simulink library "IPT_lib"  (Simulink 7.4)
settings: Solver=ode45  StartTime=0.0  StopTime=10.0  RelTol=1e-3
values from neighbouring files (symbols this model uses):
  IPTa_i_ShuntCur = mpt.Parameter    [IPT_ANALOG_CAL.m]
  IPTc_Gain_KL30 = mpt.Parameter    [IPT_ANALOG_CAL.m]
  IPTc_Gain_MSDVolt = mpt.Parameter    [IPT_ANALOG_CAL.m]
  IPTc_Gain_PCBTemp = mpt.Parameter    [IPT_ANALOG_CAL.m]
  IPTc_Gain_PosCtrVoltRef1_back = mpt.Parameter    [IPT_ANALOG_CAL.m]
  IPTc_Gain_PosCtrVoltRef1_front = mpt.Parameter    [IPT_ANALOG_CAL.m]
  IPTc_Gain_PosCtrVoltRef2_back = mpt.Parameter    [IPT_ANALOG_CAL.m]
  IPTc_Gain_PosCtrVoltRef2_front = mpt.Parameter    [IPT_ANALOG_CAL.m]
  IPTc_pct_CellInitSoc = mpt.Parameter    [IPT_INTERNAL_CAL.m]
  IPTc_t_BMUInitTemp = mpt.Parameter    [IPT_CAN_CAL.m]
  IPTc_t_MdlInitTemp = mpt.Parameter    [IPT_CAN_CAL.m]
  IPTc_t_PCBTemp_max = mpt.Parameter    [IPT_ANALOG_CAL.m]
  IPTc_t_PCBTemp_min = mpt.Parameter    [IPT_ANALOG_CAL.m]
  IPTc_v_KL30_max = mpt.Parameter    [IPT_ANALOG_CAL.m]
  IPTc_v_KL30_min = mpt.Parameter    [IPT_ANALOG_CAL.m]
  IPTc_v_MSDVolt_max = mpt.Parameter    [IPT_ANALOG_CAL.m]
  IPTc_v_MSDVolt_min = mpt.Parameter    [IPT_ANALOG_CAL.m]
  IPTc_v_PosCtrVoltRef1_back_max = mpt.Parameter    [IPT_ANALOG_CAL.m]
  IPTc_v_PosCtrVoltRef1_back_min = mpt.Parameter    [IPT_ANALOG_CAL.m]
  IPTc_v_PosCtrVoltRef1_front_max = mpt.Parameter    [IPT_ANALOG_CAL.m]
  IPTc_v_PosCtrVoltRef1_front_min = mpt.Parameter    [IPT_ANALOG_CAL.m]
  IPTc_v_PosCtrVoltRef2_back_max = mpt.Parameter    [IPT_ANALOG_CAL.m]
  IPTc_v_PosCtrVoltRef2_back_min = mpt.Parameter    [IPT_ANALOG_CAL.m]
  IPTc_v_PosCtrVoltRef2_front_max = mpt.Parameter    [IPT_ANALOG_CAL.m]
  IPTc_v_PosCtrVoltRef2_front_min = mpt.Parameter    [IPT_ANALOG_CAL.m]
  IPTf_fac_ShuntCurCorrect = mpt.Parameter    [IPT_ANALOG_CAL.m]
undefined symbols (not defined in the file or in its folder): CTC_DriveOnline_St, CTC_FastChaOnline_St, CTC_SlowChaOnline_St, IPTa_v_PCBTemp, IPTc_Gain_BMUPowSplyCur, IPTc_Gain_ShuntCur, IPTc_Gain_USample, IPTc_i_BMUPowSplyCur_max, IPTc_i_BMUPowSplyCur_min, IPTc_i_ShuntCur_max, IPTc_i_ShuntCur_min, IPTc_v_CC2_OffDnLimit, IPTc_v_CC2_OffUpLimit, IPTc_v_CC2_OnDnLimit, IPTc_v_CC2_OnUpLimit, IPTc_v_CellInitVolt, IPTc_v_SlowChalineCnctStLowLimFir, IPTc_v_SlowChalineCnctStLowLimSec, IPTc_v_SlowChalineCnctStUppLimFir, IPTc_v_SlowChalineCnctStUppLimSec, IPTc_v_SlowChalineOpenLowLim, IPTc_v_SlowChalineOpenUppLim, IPTc_v_USample_max, IPTc_v_USample_min, IPTf_t_PCBTemp, PACK_Const_BMUNumOfPack
libraries: Defined_Functionality x129
(part 1 of 3)
settings Model: Creator=zhangyanqiao  LastModifiedBy=zhouping

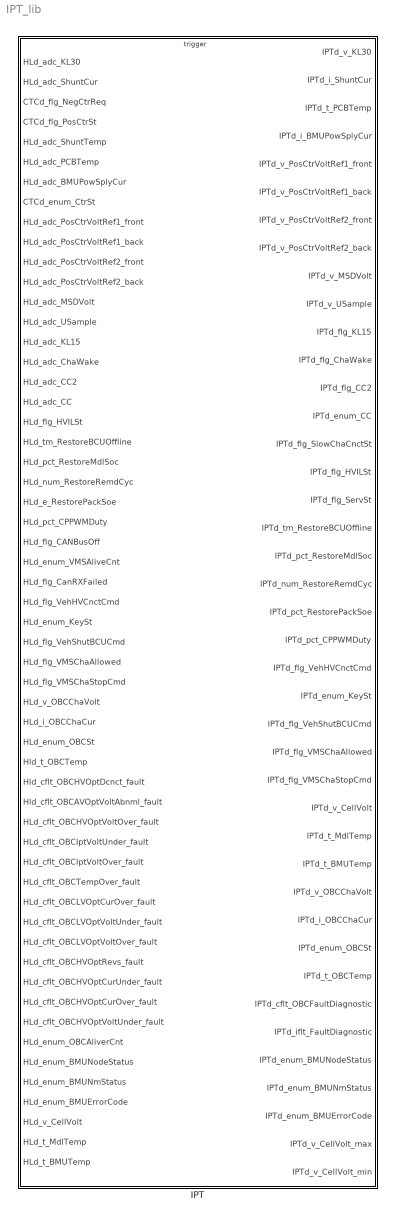
== system IPT_lib ==
  IPT : Subsystem  TreatAsAtomicUnit=on  RTWFcnName=IPT
      settings: RTWFileNameOpts=Use function name

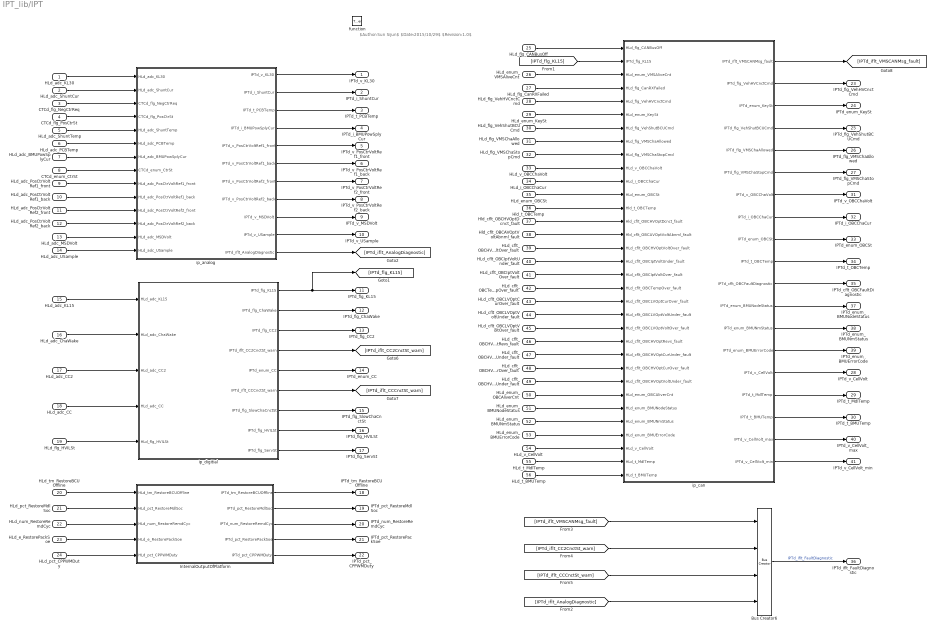
== system IPT_lib/IPT ==
  note: $Author:Sun Sijun$
      | $Date:2015/10/29$
      | $Revision:1.0$
  HLd_adc_KL30 : Inport
  HLd_adc_ShuntCur : Inport  Port=2
  CTCd_flg_NegCtrReq : Inport  Port=3
  CTCd_flg_PosCtrSt : Inport  Port=4
  HLd_adc_ShuntTemp : Inport  Port=5
  HLd_adc_PCBTemp : Inport  Port=6
  HLd_adc_BMUPowSplyCur : Inport  Port=7
  CTCd_enum_CtrSt : Inport  Port=8
  HLd_adc_PosCtrVoltRef1_front : Inport  Port=9
  HLd_adc_PosCtrVoltRef1_back : Inport  Port=10
  HLd_adc_PosCtrVoltRef2_front : Inport  Port=11
  HLd_adc_PosCtrVoltRef2_back : Inport  Port=12
  HLd_adc_MSDVolt : Inport  Port=13
  HLd_adc_USample : Inport  Port=14  OutDataType=fixdt(1, 16)  OutScaling=2^0
  HLd_adc_KL15 : Inport  Port=15
  HLd_adc_ChaWake : Inport  Port=16  OutDataType=fixdt(1, 16)  OutScaling=2^0
  HLd_adc_CC2 : Inport  Port=17  OutDataType=fixdt(1, 16)  OutScaling=2^0
  HLd_adc_CC : Inport  Port=18  OutDataType=fixdt(1, 16)  OutScaling=2^0
  HLd_flg_HVILSt : Inport  Port=19  OutDataType=fixdt(1, 16)  OutScaling=2^0
  HLd_tm_RestoreBCUOffline : Inport  Port=20  OutDataType=fixdt(1, 16)  OutScaling=2^0
  HLd_pct_RestoreMdlSoc : Inport  Port=21  OutDataType=fixdt(1, 16)  OutScaling=2^0
  HLd_num_RestoreRemdCyc : Inport  Port=22  OutDataType=fixdt(1, 16)  OutScaling=2^0
  HLd_e_RestorePackSoe : Inport  Port=23  OutDataType=fixdt(1, 16)  OutScaling=2^0
  HLd_pct_CPPWMDuty : Inport  Port=24  OutDataType=fixdt(1, 16)  OutScaling=2^0
  HLd_flg_CANBusOff : Inport  Port=25
  HLd_enum_VMSAliveCnt : Inport  Port=26  OutDataType=fixdt(1, 16)  OutScaling=2^0
  HLd_flg_CanRXFailed : Inport  Port=27  OutDataType=fixdt(1, 16)  OutScaling=2^0
  HLd_flg_VehHVCnctCmd : Inport  Port=28  OutDataType=fixdt(1, 16)  OutScaling=2^0
  HLd_enum_KeySt : Inport  Port=29  OutDataType=fixdt(1, 16)  OutScaling=2^0
  HLd_flg_VehShutBCUCmd : Inport  Port=30  OutDataType=fixdt(1, 16)  OutScaling=2^0
  HLd_flg_VMSChaAllowed : Inport  Port=31  OutDataType=fixdt(1, 16)  OutScaling=2^0
  HLd_flg_VMSChaStopCmd : Inport  Port=32  OutDataType=fixdt(1, 16)  OutScaling=2^0
  HLd_v_OBCChaVolt : Inport  Port=33
  HLd_i_OBCChaCur : Inport  Port=34
  HLd_enum_OBCSt : Inport  Port=35
  Hld_t_OBCTemp : Inport  Port=36
  Hld_cflt_OBCHVOptDcnct_fault : Inport  Port=37
  Hld_cflt_OBCAVOptVoltAbnml_fault : Inport  Port=38
  HLd_cflt_OBCHVOptVoltOver_fault : Inport  Port=39
  HLd_cflt_OBCIptVoltUnder_fault : Inport  Port=40
  HLd_cflt_OBCIptVoltOver_fault : Inport  Port=41
  HLd_cflt_OBCTempOver_fault : Inport  Port=42
  HLd_cflt_OBCLVOptCurOver_fault : Inport  Port=43
  HLd_cflt_OBCLVOptVoltUnder_fault : Inport  Port=44
  HLd_cflt_OBCLVOptVoltOver_fault : Inport  Port=45
  HLd_cflt_OBCHVOptRevs_fault : Inport  Port=46
  HLd_cflt_OBCHVOptCurUnder_fault : Inport  Port=47
  HLd_cflt_OBCHVOptCurOver_fault : Inport  Port=48
  HLd_cflt_OBCHVOptVoltUnder_fault : Inport  Port=49
  HLd_enum_OBCAliverCnt : Inport  Port=50
  HLd_enum_BMUNodeStatus : Inport  Port=51
  HLd_enum_BMUNmStatus : Inport  Port=52
  HLd_enum_BMUErrorCode : Inport  Port=53
  HLd_v_CellVolt : Inport  Port=54
  HLd_t_MdlTemp : Inport  Port=55
  HLd_t_BMUTemp : Inport  Port=56
  function : TriggerPort  TriggerType=function-call
  Bus Creator6 : BusCreator
  InternalOutputOfPlatform : Subsystem
  ip_analog : Subsystem  Description=$Author:Zhao XiangRi$
  ip_can : Subsystem
  ip_digitial : Subsystem
  IPTd_v_KL30 : Outport
  IPTd_i_ShuntCur : Outport  Port=2
  IPTd_t_PCBTemp : Outport  Port=3
  IPTd_i_BMUPowSplyCur : Outport  Port=4
  IPTd_v_PosCtrVoltRef1_front : Outport  Port=5
  IPTd_v_PosCtrVoltRef1_back : Outport  Port=6
  IPTd_v_PosCtrVoltRef2_front : Outport  Port=7
  IPTd_v_PosCtrVoltRef2_back : Outport  Port=8
  IPTd_v_MSDVolt : Outport  Port=9
  IPTd_v_USample : Outport  Port=10
  IPTd_flg_KL15 : Outport  Port=11  OutDataType=fixdt(1, 16)  OutScaling=2^0
  IPTd_flg_ChaWake : Outport  Port=12  OutDataType=fixdt(1, 16)  OutScaling=2^0
  IPTd_flg_CC2 : Outport  Port=13  OutDataType=fixdt(1, 16)  OutScaling=2^0
  IPTd_enum_CC : Outport  Port=14  OutDataType=fixdt(1, 16)  OutScaling=2^0
  IPTd_flg_SlowChaCnctSt : Outport  Port=15  OutDataType=fixdt(1, 16)  OutScaling=2^0
  IPTd_flg_HVILSt : Outport  Port=16  OutDataType=fixdt(1, 16)  OutScaling=2^0
  IPTd_flg_ServSt : Outport  Port=17  OutDataType=fixdt(1, 16)  OutScaling=2^0
  IPTd_tm_RestoreBCUOffline : Outport  Port=18  OutDataType=fixdt(1, 16)  OutScaling=2^0
  IPTd_pct_RestoreMdlSoc : Outport  Port=19  OutDataType=fixdt(1, 16)  OutScaling=2^0
  IPTd_num_RestoreRemdCyc : Outport  Port=20  OutDataType=fixdt(1, 16)  OutScaling=2^0
  IPTd_pct_RestorePackSoe : Outport  Port=21  OutDataType=fixdt(1, 16)  OutScaling=2^0
  IPTd_pct_CPPWMDuty : Outport  Port=22  OutDataType=fixdt(1, 16)  OutScaling=2^0
  IPTd_flg_VehHVCnctCmd : Outport  Port=23  OutDataType=fixdt(1, 16)  OutScaling=2^0
  IPTd_enum_KeySt : Outport  Port=24  OutDataType=fixdt(1, 16)  OutScaling=2^0
  IPTd_flg_VehShutBCUCmd : Outport  Port=25  OutDataType=fixdt(1, 16)  OutScaling=2^0
  IPTd_flg_VMSChaAllowed : Outport  Port=26  OutDataType=fixdt(1, 16)  OutScaling=2^0
  IPTd_flg_VMSChaStopCmd : Outport  Port=27  OutDataType=fixdt(1, 16)  OutScaling=2^0
  IPTd_v_CellVolt : Outport  Port=28
  IPTd_t_MdlTemp : Outport  Port=29
  IPTd_t_BMUTemp : Outport  Port=30
  IPTd_v_OBCChaVolt : Outport  Port=31
  IPTd_i_OBCChaCur : Outport  Port=32
  IPTd_enum_OBCSt : Outport  Port=33
  IPTd_t_OBCTemp : Outport  Port=34
  IPTd_cflt_OBCFaultDiagnostic : Outport  Port=35
  IPTd_iflt_FaultDiagnostic : Outport  Port=36
  "IPTd_enum_BMUNodeStatus " : Outport  Port=37
  IPTd_enum_BMUNmStatus : Outport  Port=38
  IPTd_enum_BMUErrorCode : Outport  Port=39
  IPTd_v_CellVolt_max : Outport  Port=40
  IPTd_v_CellVolt_min : Outport  Port=41
  wires:
  ip_can/19(IPTd_v_CellVolt_min) -> IPTd_v_CellVolt_min/1
  ip_can/18(IPTd_v_CellVolt_max) -> IPTd_v_CellVolt_max/1
  [IPTd_iflt_CCCnctSt_warn] -> Bus Creator6/3
  [IPTd_iflt_CC2CnctSt_warn] -> Bus Creator6/2
  ip_can/10(IPTd_t_OBCTemp) -> IPTd_t_OBCTemp/1
  Hld_cflt_OBCAVOptVoltAbnml_fault/1 -> ip_can/15(Hld_cflt_OBCAVOptVoltAbnml_fault)
  Hld_cflt_OBCHVOptDcnct_fault/1 -> ip_can/14(Hld_cflt_OBCHVOptDcnct_fault)
  Hld_t_OBCTemp/1 -> ip_can/13(Hld_t_OBCTemp)
  CTCd_flg_PosCtrSt/1 -> ip_analog/4(CTCd_flg_PosCtrSt)
  CTCd_flg_NegCtrReq/1 -> ip_analog/3(CTCd_flg_NegCtrReq)
  CTCd_enum_CtrSt/1 -> ip_analog/8(CTCd_enum_CtrSt)
  ip_digitial/9(IPTd_flg_ServSt) -> IPTd_flg_ServSt/1
  HLd_enum_BMUErrorCode/1 -> ip_can/30(HLd_enum_BMUErrorCode)
  HLd_enum_BMUNmStatus/1 -> ip_can/29(HLd_enum_BMUNmStatus)
  HLd_enum_BMUNodeStatus/1 -> ip_can/28(HLd_enum_BMUNodeStatus)
  ip_can/14(IPTd_enum_BMUErrorCode) -> IPTd_enum_BMUErrorCode/1
  ip_can/13(IPTd_enum_BMUNmStatus) -> IPTd_enum_BMUNmStatus/1
  ip_can/12("IPTd_enum_BMUNodeStatus ") -> "IPTd_enum_BMUNodeStatus "/1
  [IPTd_iflt_AnalogDiagnostic] -> Bus Creator6/4
  ip_analog/11(IPTd_iflt_AnalogDiagnostic) -> [IPTd_iflt_AnalogDiagnostic]
  ip_analog/8(IPTd_v_PosCtrVoltRef2_back) -> IPTd_v_PosCtrVoltRef2_back/1
  ip_analog/7(IPTd_v_PosCtrVoltRef2_front) -> IPTd_v_PosCtrVoltRef2_front/1
  ip_analog/6(IPTd_v_PosCtrVoltRef1_back) -> IPTd_v_PosCtrVoltRef1_back/1
  ip_analog/5(IPTd_v_PosCtrVoltRef1_front) -> IPTd_v_PosCtrVoltRef1_front/1
  ip_digitial/7(IPTd_flg_SlowChaCnctSt) -> IPTd_flg_SlowChaCnctSt/1
  ip_can/17(IPTd_t_BMUTemp) -> IPTd_t_BMUTemp/1
  HLd_t_BMUTemp/1 -> ip_can/33(HLd_t_BMUTemp)
  ip_can/11(IPTd_cflt_OBCFaultDiagnostic) -> IPTd_cflt_OBCFaultDiagnostic/1
  ip_can/9(IPTd_enum_OBCSt) -> IPTd_enum_OBCSt/1
  ip_can/8(IPTd_i_OBCChaCur) -> IPTd_i_OBCChaCur/1
  ip_can/7(IPTd_v_OBCChaVolt) -> IPTd_v_OBCChaVolt/1
  HLd_enum_OBCAliverCnt/1 -> ip_can/27(HLd_enum_OBCAliverCnt)
  HLd_cflt_OBCHVOptVoltUnder_fault/1 -> ip_can/26(HLd_cflt_OBCHVOptVoltUnder_fault)
  HLd_cflt_OBCHVOptCurOver_fault/1 -> ip_can/25(HLd_cflt_OBCHVOptCurOver_fault)
  HLd_cflt_OBCHVOptCurUnder_fault/1 -> ip_can/24(HLd_cflt_OBCHVOptCurUnder_fault)
  HLd_cflt_OBCHVOptRevs_fault/1 -> ip_can/23(HLd_cflt_OBCHVOptRevs_fault)
  HLd_cflt_OBCLVOptVoltOver_fault/1 -> ip_can/22(HLd_cflt_OBCLVOptVoltOver_fault)
  HLd_cflt_OBCLVOptVoltUnder_fault/1 -> ip_can/21(HLd_cflt_OBCLVOptVoltUnder_fault)
  HLd_cflt_OBCLVOptCurOver_fault/1 -> ip_can/20(HLd_cflt_OBCLVOptCurOver_fault)
  HLd_cflt_OBCTempOver_fault/1 -> ip_can/19(HLd_cflt_OBCTempOver_fault)
  HLd_cflt_OBCIptVoltOver_fault/1 -> ip_can/18(HLd_cflt_OBCIptVoltOver_fault)
  HLd_cflt_OBCIptVoltUnder_fault/1 -> ip_can/17(HLd_cflt_OBCIptVoltUnder_fault)
  HLd_cflt_OBCHVOptVoltOver_fault/1 -> ip_can/16(HLd_cflt_OBCHVOptVoltOver_fault)
  HLd_enum_OBCSt/1 -> ip_can/12(HLd_enum_OBCSt)
  HLd_i_OBCChaCur/1 -> ip_can/11(HLd_i_OBCChaCur)
  HLd_v_OBCChaVolt/1 -> ip_can/10(HLd_v_OBCChaVolt)
  Bus Creator6/1 -> IPTd_iflt_FaultDiagnostic/1  "IPTd_iflt_FaultDiagnostic"
  [IPTd_iflt_VMSCANMsg_fault] -> Bus Creator6/1
  ip_can/16(IPTd_t_MdlTemp) -> IPTd_t_MdlTemp/1
  ip_can/15(IPTd_v_CellVolt) -> IPTd_v_CellVolt/1
  HLd_t_MdlTemp/1 -> ip_can/32(HLd_t_MdlTemp)
  HLd_v_CellVolt/1 -> ip_can/31(HLd_v_CellVolt)
  [IPTd_flg_KL15] -> ip_can/2(IPTd_flg_KL15)
  ip_can/6(IPTd_flg_VMSChaStopCmd) -> IPTd_flg_VMSChaStopCmd/1
  ip_can/5(IPTd_flg_VMSChaAllowed) -> IPTd_flg_VMSChaAllowed/1
  ip_can/4(IPTd_flg_VehShutBCUCmd) -> IPTd_flg_VehShutBCUCmd/1
  ip_can/3(IPTd_enum_KeySt) -> IPTd_enum_KeySt/1
  ip_can/2(IPTd_flg_VehHVCnctCmd) -> IPTd_flg_VehHVCnctCmd/1
  ip_can/1(IPTd_iflt_VMSCANMsg_fault) -> [IPTd_iflt_VMSCANMsg_fault]
  HLd_flg_VMSChaStopCmd/1 -> ip_can/9(HLd_flg_VMSChaStopCmd)
  HLd_flg_VMSChaAllowed/1 -> ip_can/8(HLd_flg_VMSChaAllowed)
  HLd_flg_VehShutBCUCmd/1 -> ip_can/7(HLd_flg_VehShutBCUCmd)
  HLd_enum_KeySt/1 -> ip_can/6(HLd_enum_KeySt)
  HLd_flg_VehHVCnctCmd/1 -> ip_can/5(HLd_flg_VehHVCnctCmd)
  HLd_flg_CanRXFailed/1 -> ip_can/4(HLd_flg_CanRXFailed)
  HLd_enum_VMSAliveCnt/1 -> ip_can/3(HLd_enum_VMSAliveCnt)
  HLd_flg_CANBusOff/1 -> ip_can/1(HLd_flg_CANBusOff)
  InternalOutputOfPlatform/5(IPTd_pct_CPPWMDuty) -> IPTd_pct_CPPWMDuty/1
  HLd_pct_CPPWMDuty/1 -> InternalOutputOfPlatform/5(HLd_pct_CPPWMDuty)
  InternalOutputOfPlatform/4(IPTd_pct_RestorePackSoe) -> IPTd_pct_RestorePackSoe/1
  HLd_e_RestorePackSoe/1 -> InternalOutputOfPlatform/4(HLd_e_RestorePackSoe)
  InternalOutputOfPlatform/3(IPTd_num_RestoreRemdCyc) -> IPTd_num_RestoreRemdCyc/1
  HLd_num_RestoreRemdCyc/1 -> InternalOutputOfPlatform/3(HLd_num_RestoreRemdCyc)
  InternalOutputOfPlatform/2(IPTd_pct_RestoreMdlSoc) -> IPTd_pct_RestoreMdlSoc/1
  HLd_pct_RestoreMdlSoc/1 -> InternalOutputOfPlatform/2(HLd_pct_RestoreMdlSoc)
  InternalOutputOfPlatform/1(IPTd_tm_RestoreBCUOffline) -> IPTd_tm_RestoreBCUOffline/1
  HLd_tm_RestoreBCUOffline/1 -> InternalOutputOfPlatform/1(HLd_tm_RestoreBCUOffline)
  ip_digitial/8(IPTd_flg_HVILSt) -> IPTd_flg_HVILSt/1
  ip_digitial/6(IPTd_iflt_CCCnctSt_warn) -> [IPTd_iflt_CCCnctSt_warn]
  ip_digitial/5(IPTd_enum_CC) -> IPTd_enum_CC/1
  ip_digitial/4(IPTd_iflt_CC2CnctSt_warn) -> [IPTd_iflt_CC2CnctSt_warn]
  ip_digitial/3(IPTd_flg_CC2) -> IPTd_flg_CC2/1
  ip_analog/10(IPTd_v_USample) -> IPTd_v_USample/1
  ip_analog/9(IPTd_v_MSDVolt) -> IPTd_v_MSDVolt/1
  ip_analog/4(IPTd_i_BMUPowSplyCur) -> IPTd_i_BMUPowSplyCur/1
  ip_analog/3(IPTd_t_PCBTemp) -> IPTd_t_PCBTemp/1
  ip_analog/2(IPTd_i_ShuntCur) -> IPTd_i_ShuntCur/1
  ip_analog/1(IPTd_v_KL30) -> IPTd_v_KL30/1
  ip_digitial/2(IPTd_flg_ChaWake) -> IPTd_flg_ChaWake/1
  ip_digitial/1(IPTd_flg_KL15) -> [IPTd_flg_KL15], IPTd_flg_KL15/1
  HLd_flg_HVILSt/1 -> ip_digitial/5(HLd_flg_HVILSt)
  HLd_adc_CC/1 -> ip_digitial/4(HLd_adc_CC)
  HLd_adc_CC2/1 -> ip_digitial/3(HLd_adc_CC2)
  HLd_adc_ChaWake/1 -> ip_digitial/2(HLd_adc_ChaWake)
  HLd_adc_KL15/1 -> ip_digitial/1(HLd_adc_KL15)
  HLd_adc_MSDVolt/1 -> ip_analog/13(HLd_adc_MSDVolt)
  HLd_adc_PosCtrVoltRef2_back/1 -> ip_analog/12(HLd_adc_PosCtrVoltRef2_back)
  HLd_adc_PosCtrVoltRef2_front/1 -> ip_analog/11(HLd_adc_PosCtrVoltRef2_front)
  HLd_adc_PosCtrVoltRef1_back/1 -> ip_analog/10(HLd_adc_PosCtrVoltRef1_back)
  HLd_adc_PosCtrVoltRef1_front/1 -> ip_analog/9(HLd_adc_PosCtrVoltRef1_front)
  HLd_adc_BMUPowSplyCur/1 -> ip_analog/7(HLd_adc_BMUPowSplyCur)
  HLd_adc_PCBTemp/1 -> ip_analog/6(HLd_adc_PCBTemp)
  HLd_adc_ShuntCur/1 -> ip_analog/2(HLd_adc_ShuntCur)
  HLd_adc_KL30/1 -> ip_analog/1(HLd_adc_KL30)
  HLd_adc_ShuntTemp/1 -> ip_analog/5(HLd_adc_ShuntTemp)
  HLd_adc_USample/1 -> ip_analog/14(HLd_adc_USample)

== system IPT_lib/IPT/InternalOutputOfPlatform ==
  HLd_tm_RestoreBCUOffline : Inport  OutDataType=fixdt(1, 16)  OutScaling=2^0
  HLd_pct_RestoreMdlSoc : Inport  Port=2  OutDataType=fixdt(1, 16)  OutScaling=2^0
  HLd_num_RestoreRemdCyc : Inport  Port=3  OutDataType=fixdt(1, 16)  OutScaling=2^0
  HLd_e_RestorePackSoe : Inport  Port=4  OutDataType=fixdt(1, 16)  OutScaling=2^0
  HLd_pct_CPPWMDuty : Inport  Port=5  OutDataType=fixdt(1, 16)  OutScaling=2^0
  CPPWMDuty : Subsystem
  RestoreBCUOffline : Subsystem
  RestoreChaCycleRemained : Subsystem
  RestoreMdlSoc : Subsystem
  RestorePackSoe : Subsystem
  IPTd_tm_RestoreBCUOffline : Outport  OutDataType=fixdt(1, 16)  OutScaling=2^0
  IPTd_pct_RestoreMdlSoc : Outport  Port=2  OutDataType=fixdt(1, 16)  OutScaling=2^0
  IPTd_num_RestoreRemdCyc : Outport  Port=3  OutDataType=fixdt(1, 16)  OutScaling=2^0
  IPTd_pct_RestorePackSoe : Outport  Port=4  OutDataType=fixdt(1, 16)  OutScaling=2^0
  IPTd_pct_CPPWMDuty : Outport  Port=5  OutDataType=fixdt(1, 16)  OutScaling=2^0
  wires:
  CPPWMDuty/1(IPTd_pct_CPPWMDuty) -> IPTd_pct_CPPWMDuty/1
  HLd_pct_CPPWMDuty/1 -> CPPWMDuty/1(HLd_pct_CPPWMDuty)
  RestorePackSoe/1(IPTd_e_RestorePackSoe) -> IPTd_pct_RestorePackSoe/1
  HLd_e_RestorePackSoe/1 -> RestorePackSoe/1(HLd_e_RestorePackSoe)
  RestoreChaCycleRemained/1(IPTd_num_RestoreRemdCyc) -> IPTd_num_RestoreRemdCyc/1
  HLd_num_RestoreRemdCyc/1 -> RestoreChaCycleRemained/1(HLd_num_RestoreRemdCyc)
  RestoreMdlSoc/1(IPTd_pct_RestoreMdlSoc) -> IPTd_pct_RestoreMdlSoc/1
  HLd_pct_RestoreMdlSoc/1 -> RestoreMdlSoc/1(HLd_pct_RestoreMdlSoc)
  RestoreBCUOffline/1(IPTd_tm_RestoreBCUOffline) -> IPTd_tm_RestoreBCUOffline/1
  HLd_tm_RestoreBCUOffline/1 -> RestoreBCUOffline/1(HLd_tm_RestoreBCUOffline)

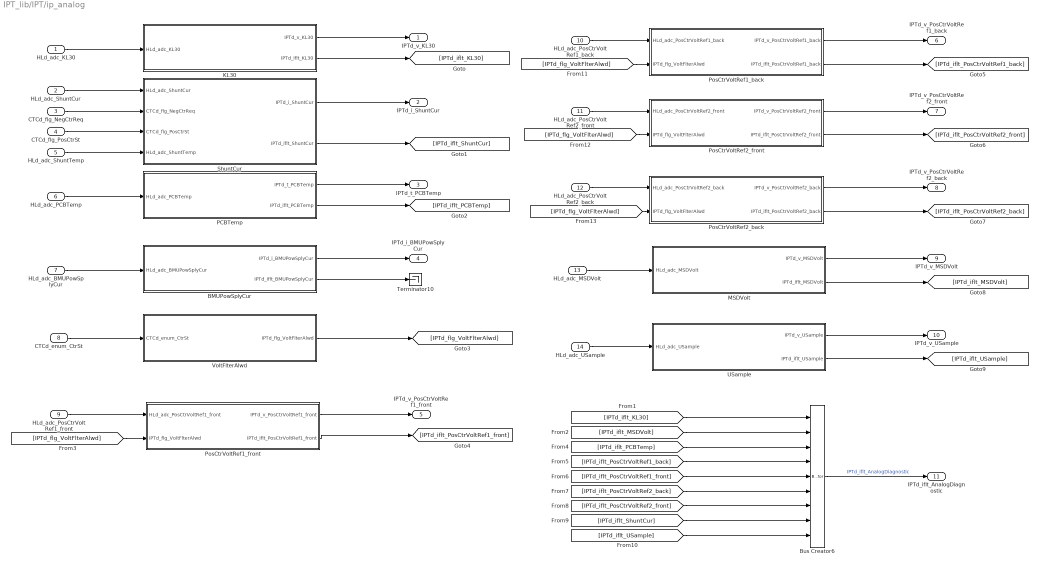
== system IPT_lib/IPT/ip_analog ==
  HLd_adc_KL30 : Inport
  HLd_adc_ShuntCur : Inport  Port=2
  CTCd_flg_NegCtrReq : Inport  Port=3
  CTCd_flg_PosCtrSt : Inport  Port=4
  HLd_adc_ShuntTemp : Inport  Port=5
  HLd_adc_PCBTemp : Inport  Port=6
  HLd_adc_BMUPowSplyCur : Inport  Port=7
  CTCd_enum_CtrSt : Inport  Port=8
  HLd_adc_PosCtrVoltRef1_front : Inport  Port=9
  HLd_adc_PosCtrVoltRef1_back : Inport  Port=10
  HLd_adc_PosCtrVoltRef2_front : Inport  Port=11
  HLd_adc_PosCtrVoltRef2_back : Inport  Port=12
  HLd_adc_MSDVolt : Inport  Port=13
  HLd_adc_USample : Inport  Port=14  OutDataType=fixdt(1, 16)  OutScaling=2^0
  BMUPowSplyCur : Subsystem  Description=$Author:Zhao XiangRi$
  Bus Creator6 : BusCreator  Inputs=9
  KL30 : Subsystem  Description=$Author:Zhao XiangRi$
  MSDVolt : Subsystem  Description=$Author:Zhao XiangRi$
  PCBTemp : Subsystem  Description=$Author:Zhao XiangRi$
  PosCtrVoltRef1_back : Subsystem  Description=$Author:Zhao XiangRi$
  PosCtrVoltRef1_front : Subsystem  Description=$Author:Zhao XiangRi$
  PosCtrVoltRef2_back : Subsystem  Description=$Author:Zhao XiangRi$
  PosCtrVoltRef2_front : Subsystem  Description=$Author:Zhao XiangRi$
  ShuntCur : Subsystem  Description=$Author:Zhao XiangRi$
  Terminator10 : Terminator
  USample : Subsystem  Description=$Author:Zhao XiangRi$
  VoltFlterAlwd : Subsystem  Description=$Author:Zhao XiangRi$
  IPTd_v_KL30 : Outport  DataType=single  OutDataTypeStr=single
  IPTd_i_ShuntCur : Outport  Port=2
  IPTd_t_PCBTemp : Outport  Port=3
  IPTd_i_BMUPowSplyCur : Outport  Port=4  DataType=single  OutDataTypeStr=single
  IPTd_v_PosCtrVoltRef1_front : Outport  Port=5
  IPTd_v_PosCtrVoltRef1_back : Outport  Port=6  DataType=single  OutDataTypeStr=single
  IPTd_v_PosCtrVoltRef2_front : Outport  Port=7  DataType=single  OutDataTypeStr=single
  IPTd_v_PosCtrVoltRef2_back : Outport  Port=8
  IPTd_v_MSDVolt : Outport  Port=9  DataType=single  OutDataTypeStr=single
  IPTd_v_USample : Outport  Port=10
  IPTd_iflt_AnalogDiagnostic : Outport  Port=11
  wires:
  CTCd_flg_PosCtrSt/1 -> ShuntCur/3(CTCd_flg_PosCtrSt)
  CTCd_flg_NegCtrReq/1 -> ShuntCur/2(CTCd_flg_NegCtrReq)
  [IPTd_flg_VoltFlterAlwd] -> PosCtrVoltRef2_back/2(IPTd_flg_VoltFlterAlwd)
  [IPTd_flg_VoltFlterAlwd] -> PosCtrVoltRef2_front/2(IPTd_flg_VoltFlterAlwd)
  [IPTd_flg_VoltFlterAlwd] -> PosCtrVoltRef1_back/2(IPTd_flg_VoltFlterAlwd)
  [IPTd_flg_VoltFlterAlwd] -> PosCtrVoltRef1_front/2(IPTd_flg_VoltFlterAlwd)
  VoltFlterAlwd/1(IPTd_flg_VoltFlterAlwd) -> [IPTd_flg_VoltFlterAlwd]
  CTCd_enum_CtrSt/1 -> VoltFlterAlwd/1(CTCd_enum_CtrSt)
  [IPTd_iflt_USample] -> Bus Creator6/9
  [IPTd_iflt_ShuntCur] -> Bus Creator6/8
  [IPTd_iflt_PosCtrVoltRef2_front] -> Bus Creator6/7
  [IPTd_iflt_PosCtrVoltRef2_back] -> Bus Creator6/6
  [IPTd_iflt_PosCtrVoltRef1_front] -> Bus Creator6/5
  [IPTd_iflt_PosCtrVoltRef1_back] -> Bus Creator6/4
  [IPTd_iflt_PCBTemp] -> Bus Creator6/3
  [IPTd_iflt_MSDVolt] -> Bus Creator6/2
  [IPTd_iflt_KL30] -> Bus Creator6/1
  Bus Creator6/1 -> IPTd_iflt_AnalogDiagnostic/1  "IPTd_iflt_AnalogDiagnostic"
  ShuntCur/2(IPTd_iflt_ShuntCur) -> [IPTd_iflt_ShuntCur]
  HLd_adc_ShuntTemp/1 -> ShuntCur/4(HLd_adc_ShuntTemp)
  PCBTemp/2(IPTd_iflt_PCBTemp) -> [IPTd_iflt_PCBTemp]
  BMUPowSplyCur/2(IPTd_iflt_BMUPowSplyCur) -> Terminator10/1
  BMUPowSplyCur/1(IPTd_i_BMUPowSplyCur) -> IPTd_i_BMUPowSplyCur/1
  KL30/2(IPTd_iflt_KL30) -> [IPTd_iflt_KL30]
  KL30/1(IPTd_v_KL30) -> IPTd_v_KL30/1
  USample/2(IPTd_iflt_USample) -> [IPTd_iflt_USample]
  MSDVolt/2(IPTd_iflt_MSDVolt) -> [IPTd_iflt_MSDVolt]
  PosCtrVoltRef2_back/2(IPTd_iflt_PosCtrVoltRef2_back) -> [IPTd_iflt_PosCtrVoltRef2_back]
  PosCtrVoltRef2_front/2(IPTd_iflt_PosCtrVoltRef2_front) -> [IPTd_iflt_PosCtrVoltRef2_front]
  PosCtrVoltRef2_front/1(IPTd_v_PosCtrVoltRef2_front) -> IPTd_v_PosCtrVoltRef2_front/1
  HLd_adc_PosCtrVoltRef2_front/1 -> PosCtrVoltRef2_front/1(HLd_adc_PosCtrVoltRef2_front)
  PosCtrVoltRef1_back/2(IPTd_iflt_PosCtrVoltRef1_back) -> [IPTd_iflt_PosCtrVoltRef1_back]
  PosCtrVoltRef1_back/1(IPTd_v_PosCtrVoltRef1_back) -> IPTd_v_PosCtrVoltRef1_back/1
  PosCtrVoltRef1_front/2(IPTd_iflt_PosCtrVoltRef1_front) -> [IPTd_iflt_PosCtrVoltRef1_front]
  USample/1(IPTd_v_USample) -> IPTd_v_USample/1
  MSDVolt/1(IPTd_v_MSDVolt) -> IPTd_v_MSDVolt/1
  PosCtrVoltRef2_back/1(IPTd_v_PosCtrVoltRef2_back) -> IPTd_v_PosCtrVoltRef2_back/1
  HLd_adc_USample/1 -> USample/1(HLd_adc_USample)
  HLd_adc_MSDVolt/1 -> MSDVolt/1(HLd_adc_MSDVolt)
  HLd_adc_PosCtrVoltRef2_back/1 -> PosCtrVoltRef2_back/1(HLd_adc_PosCtrVoltRef2_back)
  HLd_adc_PosCtrVoltRef1_back/1 -> PosCtrVoltRef1_back/1(HLd_adc_PosCtrVoltRef1_back)
  PosCtrVoltRef1_front/1(IPTd_v_PosCtrVoltRef1_front) -> IPTd_v_PosCtrVoltRef1_front/1
  HLd_adc_PosCtrVoltRef1_front/1 -> PosCtrVoltRef1_front/1(HLd_adc_PosCtrVoltRef1_front)
  PCBTemp/1(IPTd_t_PCBTemp) -> IPTd_t_PCBTemp/1
  HLd_adc_BMUPowSplyCur/1 -> BMUPowSplyCur/1(HLd_adc_BMUPowSplyCur)
  HLd_adc_PCBTemp/1 -> PCBTemp/1(HLd_adc_PCBTemp)
  ShuntCur/1(IPTd_i_ShuntCur) -> IPTd_i_ShuntCur/1
  HLd_adc_ShuntCur/1 -> ShuntCur/1(HLd_adc_ShuntCur)
  HLd_adc_KL30/1 -> KL30/1(HLd_adc_KL30)

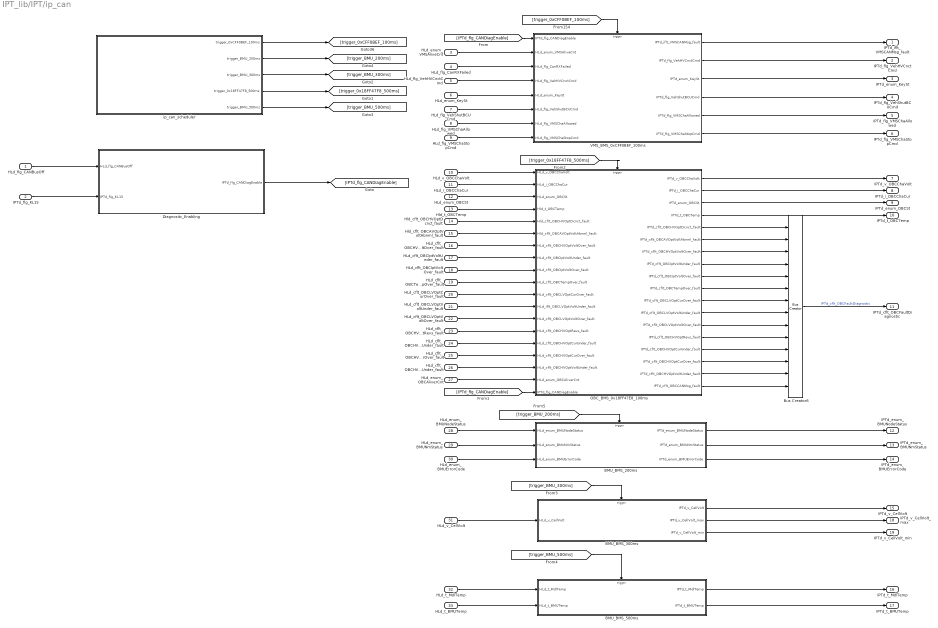
== system IPT_lib/IPT/ip_can ==
  HLd_flg_CANBusOff : Inport
  IPTd_flg_KL15 : Inport  Port=2
  HLd_enum_VMSAliveCnt : Inport  Port=3  OutDataType=fixdt(1, 16)  OutScaling=2^0
  HLd_flg_CanRXFailed : Inport  Port=4  OutDataType=fixdt(1, 16)  OutScaling=2^0
  HLd_flg_VehHVCnctCmd : Inport  Port=5  OutDataType=fixdt(1, 16)  OutScaling=2^0
  HLd_enum_KeySt : Inport  Port=6  OutDataType=fixdt(1, 16)  OutScaling=2^0
  HLd_flg_VehShutBCUCmd : Inport  Port=7  OutDataType=fixdt(1, 16)  OutScaling=2^0
  HLd_flg_VMSChaAllowed : Inport  Port=8  OutDataType=fixdt(1, 16)  OutScaling=2^0
  HLd_flg_VMSChaStopCmd : Inport  Port=9  OutDataType=fixdt(1, 16)  OutScaling=2^0
  HLd_v_OBCChaVolt : Inport  Port=10
  HLd_i_OBCChaCur : Inport  Port=11
  HLd_enum_OBCSt : Inport  Port=12
  Hld_t_OBCTemp : Inport  Port=13
  Hld_cflt_OBCHVOptDcnct_fault : Inport  Port=14
  Hld_cflt_OBCAVOptVoltAbnml_fault : Inport  Port=15
  HLd_cflt_OBCHVOptVoltOver_fault : Inport  Port=16
  HLd_cflt_OBCIptVoltUnder_fault : Inport  Port=17
  HLd_cflt_OBCIptVoltOver_fault : Inport  Port=18
  HLd_cflt_OBCTempOver_fault : Inport  Port=19
  HLd_cflt_OBCLVOptCurOver_fault : Inport  Port=20
  HLd_cflt_OBCLVOptVoltUnder_fault : Inport  Port=21
  HLd_cflt_OBCLVOptVoltOver_fault : Inport  Port=22
  HLd_cflt_OBCHVOptRevs_fault : Inport  Port=23
  HLd_cflt_OBCHVOptCurUnder_fault : Inport  Port=24
  HLd_cflt_OBCHVOptCurOver_fault : Inport  Port=25
  HLd_cflt_OBCHVOptVoltUnder_fault : Inport  Port=26
  HLd_enum_OBCAliverCnt : Inport  Port=27
  HLd_enum_BMUNodeStatus : Inport  Port=28
  HLd_enum_BMUNmStatus : Inport  Port=29
  HLd_enum_BMUErrorCode : Inport  Port=30
  HLd_v_CellVolt : Inport  Port=31
  HLd_t_MdlTemp : Inport  Port=32
  HLd_t_BMUTemp : Inport  Port=33
  BMU_BMS_200ms : Subsystem  TreatAsAtomicUnit=on
  BMU_BMS_300ms : Subsystem  TreatAsAtomicUnit=on
  BMU_BMS_500ms : Subsystem  TreatAsAtomicUnit=on
  Bus Creator6 : BusCreator  Inputs=14
  Diagnositc_Enabling : Subsystem  TreatAsAtomicUnit=on
  OBC_BMS_0x18FF47E8_100ms : Subsystem  TreatAsAtomicUnit=on
  VMS_BMS_0xCFF0BEF_100ms : Subsystem
  ip_can_scheduler : Stateflow chart  TreatAsAtomicUnit=on
  IPTd_iflt_VMSCANMsg_fault : Outport  OutDataType=fixdt(1, 16)  OutScaling=2^0
  IPTd_flg_VehHVCnctCmd : Outport  Port=2  OutDataType=fixdt(1, 16)  OutScaling=2^0
  IPTd_enum_KeySt : Outport  Port=3  OutDataType=fixdt(1, 16)  OutScaling=2^0
  IPTd_flg_VehShutBCUCmd : Outport  Port=4  OutDataType=fixdt(1, 16)  OutScaling=2^0
  IPTd_flg_VMSChaAllowed : Outport  Port=5  OutDataType=fixdt(1, 16)  OutScaling=2^0
  IPTd_flg_VMSChaStopCmd : Outport  Port=6  OutDataType=fixdt(1, 16)  OutScaling=2^0
  IPTd_v_OBCChaVolt : Outport  Port=7
  IPTd_i_OBCChaCur : Outport  Port=8
  IPTd_enum_OBCSt : Outport  Port=9
  IPTd_t_OBCTemp : Outport  Port=10
  IPTd_cflt_OBCFaultDiagnostic : Outport  Port=11
  "IPTd_enum_BMUNodeStatus " : Outport  Port=12
  IPTd_enum_BMUNmStatus : Outport  Port=13
  IPTd_enum_BMUErrorCode : Outport  Port=14
  IPTd_v_CellVolt : Outport  Port=15
  IPTd_t_MdlTemp : Outport  Port=16
  IPTd_t_BMUTemp : Outport  Port=17
  IPTd_v_CellVolt_max : Outport  Port=18
  IPTd_v_CellVolt_min : Outport  Port=19
  wires:
  BMU_BMS_300ms/3(IPTd_v_CellVolt_min) -> IPTd_v_CellVolt_min/1
  BMU_BMS_300ms/2(IPTd_v_CellVolt_max) -> IPTd_v_CellVolt_max/1
  OBC_BMS_0x18FF47E8_100ms/18(IPTd_cflt_OBCCANMsg_fault) -> Bus Creator6/14
  OBC_BMS_0x18FF47E8_100ms/17(IPTd_cflt_OBCHVOptVoltUnder_fault) -> Bus Creator6/13
  OBC_BMS_0x18FF47E8_100ms/16(IPTd_cflt_OBCHVOptCurOver_fault) -> Bus Creator6/12
  OBC_BMS_0x18FF47E8_100ms/15(IPTd_cflt_OBCHVOptCurUnder_fault) -> Bus Creator6/11
  OBC_BMS_0x18FF47E8_100ms/14(IPTd_cflt_OBCHVOptRevs_fault) -> Bus Creator6/10
  OBC_BMS_0x18FF47E8_100ms/13(IPTd_cflt_OBCLVOptVoltOver_fault) -> Bus Creator6/9
  OBC_BMS_0x18FF47E8_100ms/12(IPTd_cflt_OBCLVOptVoltUnder_fault) -> Bus Creator6/8
  OBC_BMS_0x18FF47E8_100ms/11(IPTd_cflt_OBCLVOptCurOver_fault) -> Bus Creator6/7
  OBC_BMS_0x18FF47E8_100ms/10(IPTd_cflt_OBCTempOver_fault) -> Bus Creator6/6
  OBC_BMS_0x18FF47E8_100ms/9(IPTd_cflt_OBCIptVoltOver_fault) -> Bus Creator6/5
  OBC_BMS_0x18FF47E8_100ms/8(IPTd_cflt_OBCIptVoltUnder_fault) -> Bus Creator6/4
  OBC_BMS_0x18FF47E8_100ms/7(IPTd_cflt_OBCHVOptVoltOver_fault) -> Bus Creator6/3
  OBC_BMS_0x18FF47E8_100ms/6(IPTd_cflt_OBCAVOptVoltAbnml_fault) -> Bus Creator6/2
  OBC_BMS_0x18FF47E8_100ms/5(IPTd_cflt_OBCHVOptDcnct_fault) -> Bus Creator6/1
  OBC_BMS_0x18FF47E8_100ms/4(IPTd_t_OBCTemp) -> IPTd_t_OBCTemp/1
  Hld_cflt_OBCAVOptVoltAbnml_fault/1 -> OBC_BMS_0x18FF47E8_100ms/6(Hld_cflt_OBCAVOptVoltAbnml_fault)
  Hld_cflt_OBCHVOptDcnct_fault/1 -> OBC_BMS_0x18FF47E8_100ms/5(Hld_cflt_OBCHVOptDcnct_fault)
  Hld_t_OBCTemp/1 -> OBC_BMS_0x18FF47E8_100ms/4(Hld_t_OBCTemp)
  ip_can_scheduler/2(trigger_BMU_200ms) -> [trigger_BMU_200ms]
  ip_can_scheduler/5(trigger_BMU_500ms) -> [trigger_BMU_500ms]
  ip_can_scheduler/4(trigger_0x18FF47F8_500ms) -> [trigger_0x18FF47F8_500ms]
  [trigger_BMU_200ms] -> BMU_BMS_200ms/Trigger
  BMU_BMS_200ms/3(IPTd_enum_BMUErrorCode) -> IPTd_enum_BMUErrorCode/1
  BMU_BMS_200ms/2(IPTd_enum_BMUNmStatus) -> IPTd_enum_BMUNmStatus/1
  BMU_BMS_200ms/1(IPTd_enum_BMUNodeStatus) -> "IPTd_enum_BMUNodeStatus "/1
  HLd_enum_BMUErrorCode/1 -> BMU_BMS_200ms/3(HLd_enum_BMUErrorCode)
  HLd_enum_BMUNmStatus/1 -> BMU_BMS_200ms/2(HLd_enum_BMUNmStatus)
  HLd_enum_BMUNodeStatus/1 -> BMU_BMS_200ms/1(HLd_enum_BMUNodeStatus)
  [trigger_BMU_500ms] -> BMU_BMS_500ms/Trigger
  [trigger_BMU_300ms] -> BMU_BMS_300ms/Trigger
  [trigger_0x18FF47F8_500ms] -> OBC_BMS_0x18FF47E8_100ms/Trigger
  [trigger_0xCFF0BEF_100ms] -> VMS_BMS_0xCFF0BEF_100ms/Trigger
  ip_can_scheduler/3(trigger_BMU_300ms) -> [trigger_BMU_300ms]
  ip_can_scheduler/1(trigger_0xCFF0BEF_100ms) -> [trigger_0xCFF0BEF_100ms]
  Diagnositc_Enabling/1(IPTd_flg_CANDiagEnable) -> [IPTd_flg_CANDiagEnable]
  HLd_t_MdlTemp/1 -> BMU_BMS_500ms/1(HLd_t_MdlTemp)
  BMU_BMS_500ms/2(IPTd_t_BMUTemp) -> IPTd_t_BMUTemp/1
  HLd_t_BMUTemp/1 -> BMU_BMS_500ms/2(HLd_t_BMUTemp)
  Bus Creator6/1 -> IPTd_cflt_OBCFaultDiagnostic/1  "IPTd_cflt_OBCFaultDiagnostic"
  OBC_BMS_0x18FF47E8_100ms/3(IPTd_enum_OBCSt) -> IPTd_enum_OBCSt/1
  OBC_BMS_0x18FF47E8_100ms/2(IPTd_i_OBCChaCur) -> IPTd_i_OBCChaCur/1
  OBC_BMS_0x18FF47E8_100ms/1(IPTd_v_OBCChaVolt) -> IPTd_v_OBCChaVolt/1
  [IPTd_flg_CANDiagEnable] -> OBC_BMS_0x18FF47E8_100ms/19(IPTd_flg_CANDiagEnable)
  HLd_enum_OBCAliverCnt/1 -> OBC_BMS_0x18FF47E8_100ms/18(HLd_enum_OBCAliverCnt)
  HLd_cflt_OBCHVOptVoltUnder_fault/1 -> OBC_BMS_0x18FF47E8_100ms/17(HLd_cflt_OBCHVOptVoltUnder_fault)
  HLd_cflt_OBCHVOptCurOver_fault/1 -> OBC_BMS_0x18FF47E8_100ms/16(HLd_cflt_OBCHVOptCurOver_fault)
  HLd_cflt_OBCHVOptCurUnder_fault/1 -> OBC_BMS_0x18FF47E8_100ms/15(HLd_cflt_OBCHVOptCurUnder_fault)
  HLd_cflt_OBCHVOptRevs_fault/1 -> OBC_BMS_0x18FF47E8_100ms/14(HLd_cflt_OBCHVOptRevs_fault)
  HLd_cflt_OBCLVOptVoltOver_fault/1 -> OBC_BMS_0x18FF47E8_100ms/13(HLd_cflt_OBCLVOptVoltOver_fault)
  HLd_cflt_OBCLVOptVoltUnder_fault/1 -> OBC_BMS_0x18FF47E8_100ms/12(HLd_iflt_OBCLVOptVoltUnder_fault)
  HLd_cflt_OBCLVOptCurOver_fault/1 -> OBC_BMS_0x18FF47E8_100ms/11(HLd_cflt_OBCLVOptCurOver_fault)
  HLd_cflt_OBCTempOver_fault/1 -> OBC_BMS_0x18FF47E8_100ms/10(HLd_cflt_OBCTempOver_fault)
  HLd_cflt_OBCIptVoltOver_fault/1 -> OBC_BMS_0x18FF47E8_100ms/9(HLd_cflt_OBCIptVoltOver_fault)
  HLd_cflt_OBCIptVoltUnder_fault/1 -> OBC_BMS_0x18FF47E8_100ms/8(HLd_cflt_OBCIptVoltUnder_fault)
  HLd_cflt_OBCHVOptVoltOver_fault/1 -> OBC_BMS_0x18FF47E8_100ms/7(HLd_cflt_OBCHVOptVoltOver_fault)
  HLd_enum_OBCSt/1 -> OBC_BMS_0x18FF47E8_100ms/3(HLd_enum_OBCSt)
  HLd_i_OBCChaCur/1 -> OBC_BMS_0x18FF47E8_100ms/2(HLd_i_OBCChaCur)
  HLd_v_OBCChaVolt/1 -> OBC_BMS_0x18FF47E8_100ms/1(HLd_v_OBCChaVolt)
  VMS_BMS_0xCFF0BEF_100ms/6(IPTd_flg_VMSChaStopCmd) -> IPTd_flg_VMSChaStopCmd/1
  VMS_BMS_0xCFF0BEF_100ms/4(IPTd_flg_VehShutBCUCmd) -> IPTd_flg_VehShutBCUCmd/1
  VMS_BMS_0xCFF0BEF_100ms/3(IPTd_enum_KeySt) -> IPTd_enum_KeySt/1
  VMS_BMS_0xCFF0BEF_100ms/2(IPTd_flg_VehHVCnctCmd) -> IPTd_flg_VehHVCnctCmd/1
  BMU_BMS_500ms/1(IPTd_t_MdlTemp) -> IPTd_t_MdlTemp/1
  BMU_BMS_300ms/1(IPTd_v_CellVolt) -> IPTd_v_CellVolt/1
  HLd_v_CellVolt/1 -> BMU_BMS_300ms/1(HLd_v_CellVolt)
  IPTd_flg_KL15/1 -> Diagnositc_Enabling/2(IPTd_flg_KL15)
  HLd_flg_CANBusOff/1 -> Diagnositc_Enabling/1(HLd_flg_CANBusOff)
  VMS_BMS_0xCFF0BEF_100ms/5(IPTd_flg_VMSChaAllowed) -> IPTd_flg_VMSChaAllowed/1
  VMS_BMS_0xCFF0BEF_100ms/1(IPTd_iflt_VMSCANMsg_fault) -> IPTd_iflt_VMSCANMsg_fault/1
  HLd_flg_VMSChaStopCmd/1 -> VMS_BMS_0xCFF0BEF_100ms/8(HLd_flg_VMSChaStopCmd)
  HLd_flg_VMSChaAllowed/1 -> VMS_BMS_0xCFF0BEF_100ms/7(HLd_flg_VMSChaAllowed)
  HLd_flg_VehShutBCUCmd/1 -> VMS_BMS_0xCFF0BEF_100ms/6(HLd_flg_VehShutBCUCmd)
  HLd_enum_KeySt/1 -> VMS_BMS_0xCFF0BEF_100ms/5(HLd_enum_KeySt)
  HLd_flg_VehHVCnctCmd/1 -> VMS_BMS_0xCFF0BEF_100ms/4(HLd_flg_VehHVCnctCmd)
  HLd_flg_CanRXFailed/1 -> VMS_BMS_0xCFF0BEF_100ms/3(HLd_flg_CanRXFailed)
  HLd_enum_VMSAliveCnt/1 -> VMS_BMS_0xCFF0BEF_100ms/2(HLd_enum_VMSAliveCnt)
  [IPTd_flg_CANDiagEnable] -> VMS_BMS_0xCFF0BEF_100ms/1(IPTd_flg_CANDiagEnable)

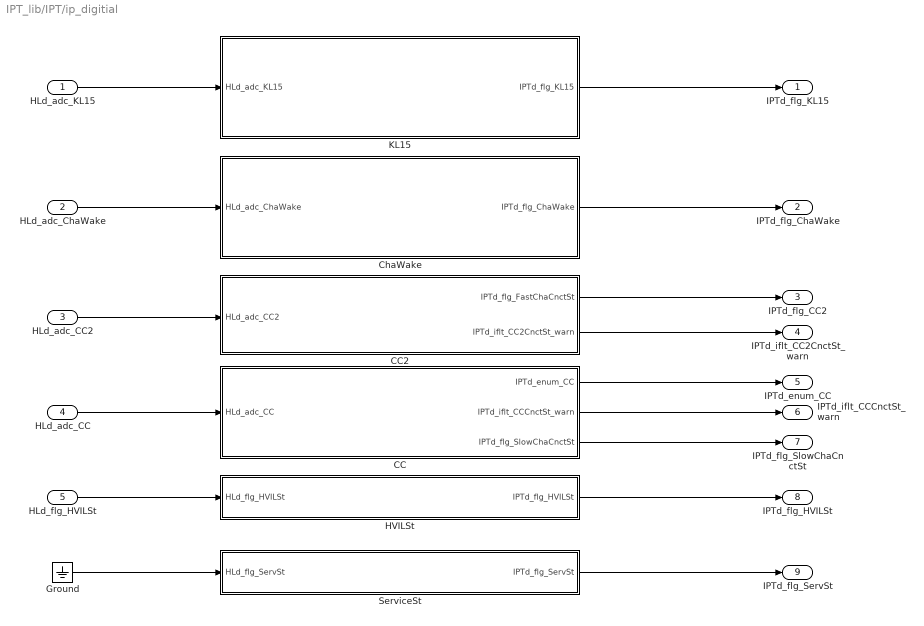
== system IPT_lib/IPT/ip_digitial ==
  HLd_adc_KL15 : Inport  OutDataType=fixdt(1, 16)  OutScaling=2^0
  HLd_adc_ChaWake : Inport  Port=2  OutDataType=fixdt(1, 16)  OutScaling=2^0
  HLd_adc_CC2 : Inport  Port=3  OutDataType=fixdt(1, 16)  OutScaling=2^0
  HLd_adc_CC : Inport  Port=4  OutDataType=fixdt(1, 16)  OutScaling=2^0
  HLd_flg_HVILSt : Inport  Port=5  OutDataType=fixdt(1, 16)  OutScaling=2^0
  CC : Subsystem
  CC2 : Subsystem
  ChaWake : Subsystem
  Ground : Ground
  HVILSt : Subsystem
  KL15 : Subsystem
  ServiceSt : Subsystem
  IPTd_flg_KL15 : Outport  OutDataType=fixdt(1, 16)  OutScaling=2^0
  IPTd_flg_ChaWake : Outport  Port=2  OutDataType=fixdt(1, 16)  OutScaling=2^0
  IPTd_flg_CC2 : Outport  Port=3  OutDataType=fixdt(1, 16)  OutScaling=2^0
  IPTd_iflt_CC2CnctSt_warn : Outport  Port=4  OutDataType=fixdt(1, 16)  OutScaling=2^0
  IPTd_enum_CC : Outport  Port=5  OutDataType=fixdt(1, 16)  OutScaling=2^0
  IPTd_iflt_CCCnctSt_warn : Outport  Port=6  OutDataType=fixdt(1, 16)  OutScaling=2^0
  IPTd_flg_SlowChaCnctSt : Outport  Port=7  OutDataType=fixdt(1, 16)  OutScaling=2^0
  IPTd_flg_HVILSt : Outport  Port=8  OutDataType=fixdt(1, 16)  OutScaling=2^0
  IPTd_flg_ServSt : Outport  Port=9  OutDataType=fixdt(1, 16)  OutScaling=2^0
  wires:
  CC/3(IPTd_flg_SlowChaCnctSt) -> IPTd_flg_SlowChaCnctSt/1
  HVILSt/1(IPTd_flg_HVILSt) -> IPTd_flg_HVILSt/1
  CC/2(IPTd_iflt_CCCnctSt_warn) -> IPTd_iflt_CCCnctSt_warn/1
  CC/1(IPTd_enum_CC) -> IPTd_enum_CC/1
  CC2/2(IPTd_iflt_CC2CnctSt_warn) -> IPTd_iflt_CC2CnctSt_warn/1
  CC2/1(IPTd_flg_FastChaCnctSt) -> IPTd_flg_CC2/1
  ChaWake/1(IPTd_flg_ChaWake) -> IPTd_flg_ChaWake/1
  KL15/1(IPTd_flg_KL15) -> IPTd_flg_KL15/1
  HLd_flg_HVILSt/1 -> HVILSt/1(HLd_flg_HVILSt)
  HLd_adc_CC/1 -> CC/1(HLd_adc_CC)
  HLd_adc_CC2/1 -> CC2/1(HLd_adc_CC2)
  HLd_adc_ChaWake/1 -> ChaWake/1(HLd_adc_ChaWake)
  HLd_adc_KL15/1 -> KL15/1(HLd_adc_KL15)
  ServiceSt/1(IPTd_flg_ServSt) -> IPTd_flg_ServSt/1
  Ground/1 -> ServiceSt/1(HLd_flg_ServSt)

== system IPT_lib/IPT/InternalOutputOfPlatform/CPPWMDuty ==
  HLd_pct_CPPWMDuty : Inport  OutDataType=fixdt(1, 16)  OutScaling=2^0
  saturation4 : Defined_Functionality/saturation  SystemSampleTime=-1  upper_limit=1  lower_limit=0
      settings: AttributesFormatString=[UPPER_LIMIT=%<upper_limit>]\n[LOWER_LIMIT=%<lower_limit>]
  signal_debug5 : Defined_Functionality/signal_debug  SystemSampleTime=-1  debug_switch=IPTc_dbgsw_pct_CPPWMDuty  debug_value=IPTc_dbgval_pct_CPPWMDuty
      settings: AttributesFormatString=[SWITCH=%<debug_switch>]\n[VALUE=%<debug_value>]
  IPTd_pct_CPPWMDuty : Outport  OutDataType=fixdt(1, 16)  OutScaling=2^0
  wires:
  saturation4/1 -> signal_debug5/1
  signal_debug5/1 -> IPTd_pct_CPPWMDuty/1  "IPTd_pct_CPPWMDuty"
  HLd_pct_CPPWMDuty/1 -> saturation4/1

== system IPT_lib/IPT/InternalOutputOfPlatform/RestoreBCUOffline ==
  HLd_tm_RestoreBCUOffline : Inport  OutDataType=fixdt(1, 16)  OutScaling=2^0
  saturation3 : Defined_Functionality/saturation  SystemSampleTime=-1  upper_limit=65536  lower_limit=0
      settings: AttributesFormatString=[UPPER_LIMIT=%<upper_limit>]\n[LOWER_LIMIT=%<lower_limit>]
  signal_debug : Defined_Functionality/signal_debug  SystemSampleTime=-1  debug_switch=IPTc_dbgsw_tm_BCUOffline  debug_value=IPTc_dbgval_tm_BCUOffline
      settings: AttributesFormatString=[SWITCH=%<debug_switch>]\n[VALUE=%<debug_value>]
  IPTd_tm_RestoreBCUOffline : Outport  OutDataType=fixdt(1, 16)  OutScaling=2^0
  wires:
  saturation3/1 -> signal_debug/1
  signal_debug/1 -> IPTd_tm_RestoreBCUOffline/1  "IPTd_tm_RestoreBCUOffline"
  HLd_tm_RestoreBCUOffline/1 -> saturation3/1

== system IPT_lib/IPT/InternalOutputOfPlatform/RestoreChaCycleRemained ==
  HLd_num_RestoreRemdCyc : Inport  OutDataType=fixdt(1, 16)  OutScaling=2^0
  CAN to Actual Value : Defined_Functionality/CAN to Actual Value  SystemSampleTime=-1  gain=0.1  offset=0
      settings: AttributesFormatString=[GAIN=%<gain>]\n[OFFSET=%<offset>]
  saturation2 : Defined_Functionality/saturation  SystemSampleTime=-1  upper_limit=5000  lower_limit=0
      settings: AttributesFormatString=[UPPER_LIMIT=%<upper_limit>]\n[LOWER_LIMIT=%<lower_limit>]
  signal_debug2 : Defined_Functionality/signal_debug  SystemSampleTime=-1  debug_switch=IPTc_dbgsw_RestoreChaCycle  debug_value=IPTc_dbgval_RestoreChaCycle
      settings: AttributesFormatString=[SWITCH=%<debug_switch>]\n[VALUE=%<debug_value>]
  IPTd_num_RestoreRemdCyc : Outport  OutDataType=fixdt(1, 16)  OutScaling=2^0
  wires:
  CAN to Actual Value/1 -> saturation2/1
  saturation2/1 -> signal_debug2/1
  HLd_num_RestoreRemdCyc/1 -> CAN to Actual Value/1
  signal_debug2/1 -> IPTd_num_RestoreRemdCyc/1  "IPTd_num_RestoreRemdCyc"

== system IPT_lib/IPT/InternalOutputOfPlatform/RestoreMdlSoc ==
  HLd_pct_RestoreMdlSoc : Inport  OutDataType=fixdt(1, 16)  OutScaling=2^0
  CellSoc : Subsystem  TreatAsAtomicUnit=on
  signal_debug : Defined_Functionality/signal_debug  SystemSampleTime=-1  debug_switch=IPTc_dbgsw_pct_RestoreCellSoc  debug_value=IPTc_dbgval_RestoreCellSoc
      settings: AttributesFormatString=[SWITCH=%<debug_switch>]\n[VALUE=%<debug_value>]
  IPTd_pct_RestoreMdlSoc : Outport  OutDataType=fixdt(1, 16)  OutScaling=2^0
  wires:
  signal_debug/1 -> IPTd_pct_RestoreMdlSoc/1  "IPTd_pct_RestoreMdlSoc"
  CellSoc/1(CellMdlOut) -> signal_debug/1
  HLd_pct_RestoreMdlSoc/1 -> CellSoc/1(CellMdlIn)

== system IPT_lib/IPT/InternalOutputOfPlatform/RestorePackSoe ==
  HLd_e_RestorePackSoe : Inport  OutDataType=fixdt(1, 16)  OutScaling=2^0
  CAN to Actual Value : Defined_Functionality/CAN to Actual Value  SystemSampleTime=-1  gain=0.01  offset=0
      settings: AttributesFormatString=[GAIN=%<gain>]\n[OFFSET=%<offset>]
  saturation1 : Defined_Functionality/saturation  SystemSampleTime=-1  upper_limit=300  lower_limit=0
      settings: AttributesFormatString=[UPPER_LIMIT=%<upper_limit>]\n[LOWER_LIMIT=%<lower_limit>]
  signal_debug3 : Defined_Functionality/signal_debug  SystemSampleTime=-1  debug_switch=IPTc_dbgsw_e_PackSoe  debug_value=IPTc_dbgval_e_PackSoe
      settings: AttributesFormatString=[SWITCH=%<debug_switch>]\n[VALUE=%<debug_value>]
  IPTd_e_RestorePackSoe : Outport  OutDataType=fixdt(1, 16)  OutScaling=2^0
  wires:
  CAN to Actual Value/1 -> saturation1/1
  saturation1/1 -> signal_debug3/1
  signal_debug3/1 -> IPTd_e_RestorePackSoe/1  "IPTd_e_RestorePackSoe"
  HLd_e_RestorePackSoe/1 -> CAN to Actual Value/1

== system IPT_lib/IPT/ip_analog/BMUPowSplyCur ==
  HLd_adc_BMUPowSplyCur : Inport
  ADC to Actual Value1 : Defined_Functionality/ADC to Actual Value1  SystemSampleTime=-1  offset=IPTc_Offset_BMUPowSplyCur  gain=IPTc_Gain_BMUPowSplyCur
      settings: AttributesFormatString=[OFFSET=%<offset>]\n[GAIN=%<gain>]
  Constant : Constant  Value=IPTc_i_BMUPowSplyCur_max  OutDataTypeMode=single  OutDataType=fixdt(1, 16)  OutScaling=2^0  OutDataTypeStr=single
  Constant1 : Constant  Value=IPTc_i_BMUPowSplyCur_min  OutDataTypeMode=single  OutDataType=fixdt(1, 16)  OutScaling=2^0  OutDataTypeStr=single
  LPF1 : Defined_Functionality/LPF  SystemSampleTime=-1  filter_gain=IPTc_flter_BMUPowSplyCur
      settings: AttributesFormatString=[FILTER_GAIN=%<filter_gain>]
  Logical Operator : Logic  Operator=OR  AllPortsSameDT=off  OutDataTypeMode=boolean  LogicDataType=fixdt(0, 8)  OutDataTypeStr=boolean
  Relational Operator : RelationalOperator  Operator=>  LogicOutDataTypeMode=boolean  LogicDataType=fixdt(0, 8)  OutDataTypeStr=boolean
  Relational Operator1 : RelationalOperator  Operator=<  LogicOutDataTypeMode=boolean  LogicDataType=fixdt(0, 8)  OutDataTypeStr=boolean
  saturation : Defined_Functionality/saturation  SystemSampleTime=-1  upper_limit=IPTc_i_BMUPowSplyCur_max  lower_limit=IPTc_i_BMUPowSplyCur_min
      settings: AttributesFormatString=[UPPER_LIMIT=%<upper_limit>]\n[LOWER_LIMIT=%<lower_limit>]
  signal_debug : Defined_Functionality/signal_debug  SystemSampleTime=-1  debug_switch=IPTc_dbgsw_BMUPowSplyCur  debug_value=IPTc_dbgval_BMUPowSplyCur
  IPTd_i_BMUPowSplyCur : Outport
  IPTd_iflt_BMUPowSplyCur : Outport  Port=2
  wires:
  ADC to Actual Value1/1 -> LPF1/1  "IPTd_v_BMUPowSplyCur_raw"
  Relational Operator1/1 -> Logical Operator/2
  Relational Operator/1 -> Logical Operator/1
  Constant1/1 -> Relational Operator1/2
  Constant/1 -> Relational Operator/2
  saturation/1 -> signal_debug/1
  signal_debug/1 -> IPTd_i_BMUPowSplyCur/1  "IPTd_i_BMUPowSplyCur"
  Logical Operator/1 -> IPTd_iflt_BMUPowSplyCur/1  "IPTd_iflt_BMUPowSplyCur"
  LPF1/1 -> Relational Operator1/1, Relational Operator/1, saturation/1
  HLd_adc_BMUPowSplyCur/1 -> ADC to Actual Value1/1

== system IPT_lib/IPT/ip_analog/KL30 ==
  HLd_adc_KL30 : Inport
  ADC to Actual Value2 : Defined_Functionality/ADC to Actual Value1  SystemSampleTime=-1  offset=IPTc_Offset_KL30  gain=IPTc_Gain_KL30
      settings: AttributesFormatString=[OFFSET=%<offset>]\n[GAIN=%<gain>]
  Constant : Constant  Value=IPTc_v_KL30_max  OutDataTypeMode=single  OutDataType=fixdt(1, 16)  OutScaling=2^0  OutDataTypeStr=single
  Constant1 : Constant  Value=IPTc_v_KL30_min  OutDataTypeMode=single  OutDataType=fixdt(1, 16)  OutScaling=2^0  OutDataTypeStr=single
  LPF1 : Defined_Functionality/LPF  SystemSampleTime=-1  filter_gain=IPTc_flter_KL30
      settings: AttributesFormatString=[FILTER_GAIN=%<filter_gain>]
  Logical Operator : Logic  Operator=OR  AllPortsSameDT=off  OutDataTypeMode=boolean  LogicDataType=fixdt(0, 8)  OutDataTypeStr=boolean
  Relational Operator : RelationalOperator  Operator=>  LogicOutDataTypeMode=boolean  LogicDataType=fixdt(0, 8)  OutDataTypeStr=boolean
  Relational Operator1 : RelationalOperator  Operator=<  LogicOutDataTypeMode=boolean  LogicDataType=fixdt(0, 8)  OutDataTypeStr=boolean
  saturation : Defined_Functionality/saturation  SystemSampleTime=-1  upper_limit=IPTc_v_KL30_max  lower_limit=0
      settings: AttributesFormatString=[UPPER_LIMIT=%<upper_limit>]\n[LOWER_LIMIT=%<lower_limit>]
  signal_debug : Defined_Functionality/signal_debug  SystemSampleTime=-1  debug_switch=IPTc_dbgsw_KL30  debug_value=IPTc_dbgval_KL30
  IPTd_v_KL30 : Outport
  IPTd_iflt_KL30 : Outport  Port=2
  wires:
  ADC to Actual Value2/1 -> LPF1/1  "IPTd_v_KL30_raw"
  Relational Operator/1 -> Logical Operator/1
  Constant/1 -> Relational Operator/2
  Constant1/1 -> Relational Operator1/2
  Relational Operator1/1 -> Logical Operator/2
  saturation/1 -> signal_debug/1
  HLd_adc_KL30/1 -> ADC to Actual Value2/1
  LPF1/1 -> Relational Operator/1, Relational Operator1/1, saturation/1
  Logical Operator/1 -> IPTd_iflt_KL30/1  "IPTd_iflt_KL30"
  signal_debug/1 -> IPTd_v_KL30/1  "IPTd_v_KL30"

== system IPT_lib/IPT/ip_analog/MSDVolt ==
  HLd_adc_MSDVolt : Inport
  ADC to Actual Value1 : Defined_Functionality/ADC to Actual Value1  SystemSampleTime=-1  offset=IPTc_Offset_MSDVolt  gain=IPTc_Gain_MSDVolt
      settings: AttributesFormatString=[OFFSET=%<offset>]\n[GAIN=%<gain>]
  Constant : Constant  Value=IPTc_v_MSDVolt_max  OutDataTypeMode=single  OutDataType=fixdt(1, 16)  OutScaling=2^0  OutDataTypeStr=single
  Constant1 : Constant  Value=IPTc_v_MSDVolt_min  OutDataTypeMode=single  OutDataType=fixdt(1, 16)  OutScaling=2^0  OutDataTypeStr=single
  LPF1 : Defined_Functionality/LPF  SystemSampleTime=-1  filter_gain=IPTc_flter_MSDVolt
      settings: AttributesFormatString=[FILTER_GAIN=%<filter_gain>]
  Logical Operator : Logic  Operator=OR  AllPortsSameDT=off  OutDataTypeMode=boolean  LogicDataType=fixdt(0, 8)  OutDataTypeStr=boolean
  Relational Operator : RelationalOperator  Operator=>  LogicOutDataTypeMode=boolean  LogicDataType=fixdt(0, 8)  OutDataTypeStr=boolean
  Relational Operator1 : RelationalOperator  Operator=<  LogicOutDataTypeMode=boolean  LogicDataType=fixdt(0, 8)  OutDataTypeStr=boolean
  saturation : Defined_Functionality/saturation  SystemSampleTime=-1  upper_limit=IPTc_v_MSDVolt_max  lower_limit=IPTc_v_MSDVolt_min
      settings: AttributesFormatString=[UPPER_LIMIT=%<upper_limit>]\n[LOWER_LIMIT=%<lower_limit>]
  signal_debug : Defined_Functionality/signal_debug  SystemSampleTime=-1  debug_switch=IPTc_dbgsw_MSDVolt  debug_value=IPTc_dbgval_MSDVolt
  IPTd_v_MSDVolt : Outport  DataType=single  OutDataTypeStr=single
  IPTd_iflt_MSDVolt : Outport  Port=2
  wires:
  ADC to Actual Value1/1 -> LPF1/1  "IPTd_v_MSDVolt_raw"
  LPF1/1 -> Relational Operator1/1, Relational Operator/1, saturation/1
  Relational Operator1/1 -> Logical Operator/2
  Relational Operator/1 -> Logical Operator/1
  Constant1/1 -> Relational Operator1/2
  Constant/1 -> Relational Operator/2
  saturation/1 -> signal_debug/1
  signal_debug/1 -> IPTd_v_MSDVolt/1  "IPTd_v_MSDVolt"
  Logical Operator/1 -> IPTd_iflt_MSDVolt/1  "IPTd_iflt_MSDVolt"
  HLd_adc_MSDVolt/1 -> ADC to Actual Value1/1

== system IPT_lib/IPT/ip_analog/PCBTemp ==
  HLd_adc_PCBTemp : Inport
  Constant : Constant  Value=IPTc_t_PCBTemp_max  OutDataTypeMode=single  OutDataType=fixdt(1, 16)  OutScaling=2^0  OutDataTypeStr=single
  Constant1 : Constant  Value=IPTc_t_PCBTemp_min  OutDataTypeMode=single  OutDataType=fixdt(1, 16)  OutScaling=2^0  OutDataTypeStr=single
  Conversion : Subsystem  Description=$Author:Zhao XiangRi$
  LPF1 : Defined_Functionality/LPF  SystemSampleTime=-1  filter_gain=IPTc_flter_PCBTemp
      settings: AttributesFormatString=[FILTER_GAIN=%<filter_gain>]
  Logical Operator : Logic  Operator=OR  AllPortsSameDT=off  OutDataTypeMode=boolean  LogicDataType=fixdt(0, 8)  OutDataTypeStr=boolean
  Relational Operator : RelationalOperator  Operator=>  LogicOutDataTypeMode=boolean  LogicDataType=fixdt(0, 8)  OutDataTypeStr=boolean
  Relational Operator1 : RelationalOperator  Operator=<  LogicOutDataTypeMode=boolean  LogicDataType=fixdt(0, 8)  OutDataTypeStr=boolean
  saturation : Defined_Functionality/saturation  SystemSampleTime=-1  upper_limit=IPTc_t_PCBTemp_max  lower_limit=IPTc_t_PCBTemp_min
      settings: AttributesFormatString=[UPPER_LIMIT=%<upper_limit>]\n[LOWER_LIMIT=%<lower_limit>]
  signal_debug : Defined_Functionality/signal_debug  SystemSampleTime=-1  debug_switch=IPTc_dbgsw_PCBTemp  debug_value=IPTc_dbgval_PCBTemp
  IPTd_t_PCBTemp : Outport
  IPTd_iflt_PCBTemp : Outport  Port=2
  wires:
  saturation/1 -> signal_debug/1
  Constant/1 -> Relational Operator/2
  Constant1/1 -> Relational Operator1/2
  Relational Operator/1 -> Logical Operator/1
  Relational Operator1/1 -> Logical Operator/2
  HLd_adc_PCBTemp/1 -> Conversion/1(ADC)
  Conversion/1(Volt) -> LPF1/1
  LPF1/1 -> Relational Operator1/1, Relational Operator/1, saturation/1
  Logical Operator/1 -> IPTd_iflt_PCBTemp/1  "IPTd_iflt_PCBTemp"
  signal_debug/1 -> IPTd_t_PCBTemp/1  "IPTd_t_PCBTemp"

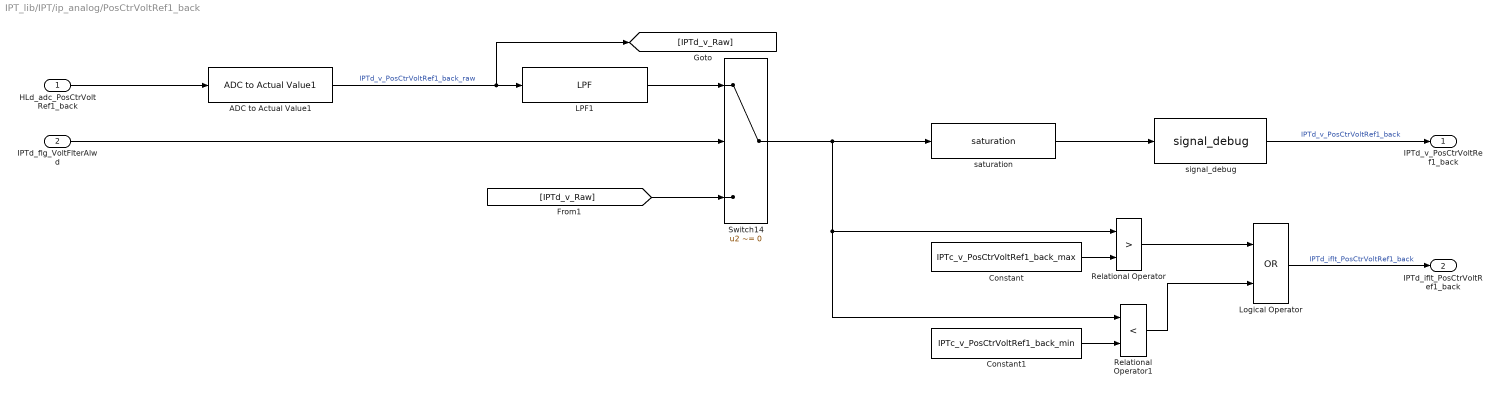
== system IPT_lib/IPT/ip_analog/PosCtrVoltRef1_back ==
  HLd_adc_PosCtrVoltRef1_back : Inport
  IPTd_flg_VoltFlterAlwd : Inport  Port=2
  ADC to Actual Value1 : Defined_Functionality/ADC to Actual Value1  SystemSampleTime=-1  offset=IPTc_Offset_PosCtrVoltRef1_back  gain=IPTc_Gain_PosCtrVoltRef1_back
      settings: AttributesFormatString=[OFFSET=%<offset>]\n[GAIN=%<gain>]
  Constant : Constant  Value=IPTc_v_PosCtrVoltRef1_back_max  OutDataTypeMode=single  OutDataType=fixdt(1, 16)  OutScaling=2^0  OutDataTypeStr=single
  Constant1 : Constant  Value=IPTc_v_PosCtrVoltRef1_back_min  OutDataTypeMode=single  OutDataType=fixdt(1, 16)  OutScaling=2^0  OutDataTypeStr=single
  LPF1 : Defined_Functionality/LPF  SystemSampleTime=-1  filter_gain=IPTc_flter_PosCtrVoltRef1_back
      settings: AttributesFormatString=[FILTER_GAIN=%<filter_gain>]
  Logical Operator : Logic  Operator=OR  AllPortsSameDT=off  OutDataTypeMode=boolean  LogicDataType=fixdt(0, 8)  OutDataTypeStr=boolean
  Relational Operator : RelationalOperator  Operator=>  LogicOutDataTypeMode=boolean  LogicDataType=fixdt(0, 8)  OutDataTypeStr=boolean
  Relational Operator1 : RelationalOperator  Operator=<  LogicOutDataTypeMode=boolean  LogicDataType=fixdt(0, 8)  OutDataTypeStr=boolean
  Switch14 : Switch  Criteria=u2 ~= 0  Threshold=0.5  OutDataTypeMode=single  OutDataType=sfix(16)  OutScaling=2^0  OutDataTypeStr=single
  saturation : Defined_Functionality/saturation  SystemSampleTime=-1  upper_limit=IPTc_v_PosCtrVoltRef1_back_max  lower_limit=IPTc_v_PosCtrVoltRef1_back_min
      settings: AttributesFormatString=[UPPER_LIMIT=%<upper_limit>]\n[LOWER_LIMIT=%<lower_limit>]
  signal_debug : Defined_Functionality/signal_debug  SystemSampleTime=-1  debug_switch=IPTc_dbgsw_PosCtrVoltRef1_back  debug_value=IPTc_dbgval_PosCtrVoltRef1_back
  IPTd_v_PosCtrVoltRef1_back : Outport
  IPTd_iflt_PosCtrVoltRef1_back : Outport  Port=2
  wires:
  ADC to Actual Value1/1 -> [IPTd_v_Raw], LPF1/1  "IPTd_v_PosCtrVoltRef1_back_raw"
  Switch14/1 -> Relational Operator1/1, Relational Operator/1, saturation/1
  LPF1/1 -> Switch14/1
  [IPTd_v_Raw] -> Switch14/3
  IPTd_flg_VoltFlterAlwd/1 -> Switch14/2
  Relational Operator1/1 -> Logical Operator/2
  Relational Operator/1 -> Logical Operator/1
  Constant1/1 -> Relational Operator1/2
  Constant/1 -> Relational Operator/2
  saturation/1 -> signal_debug/1
  signal_debug/1 -> IPTd_v_PosCtrVoltRef1_back/1  "IPTd_v_PosCtrVoltRef1_back"
  Logical Operator/1 -> IPTd_iflt_PosCtrVoltRef1_back/1  "IPTd_iflt_PosCtrVoltRef1_back"
  HLd_adc_PosCtrVoltRef1_back/1 -> ADC to Actual Value1/1
